simulink model "TaskB"  (R2022b)
settings: Solver=ode45  StartTime=0.0  StopTime=10.0  RelTol=1e-3
undefined symbols (not defined in the file): A_11, A_12, A_21, A_22, absolute_encoder_counts_per_revolution, B_1, B_2, init, K_I2, K_x2, L_d
libraries: simulink_extras x7
settings Model: Creator=tumisangramotlhwa  LastModifiedBy=tumisangramotlhwa

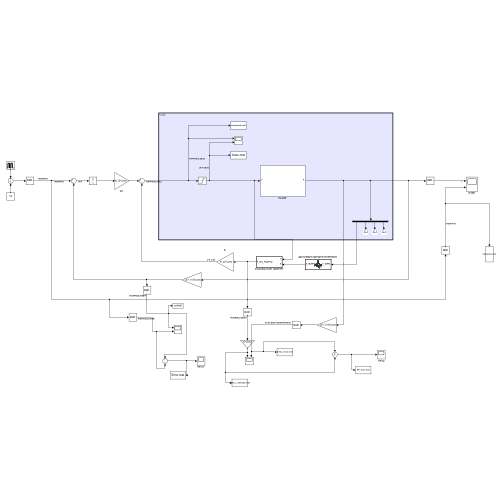
[thumbnail: Simulink's stored preview of the top-level diagram]
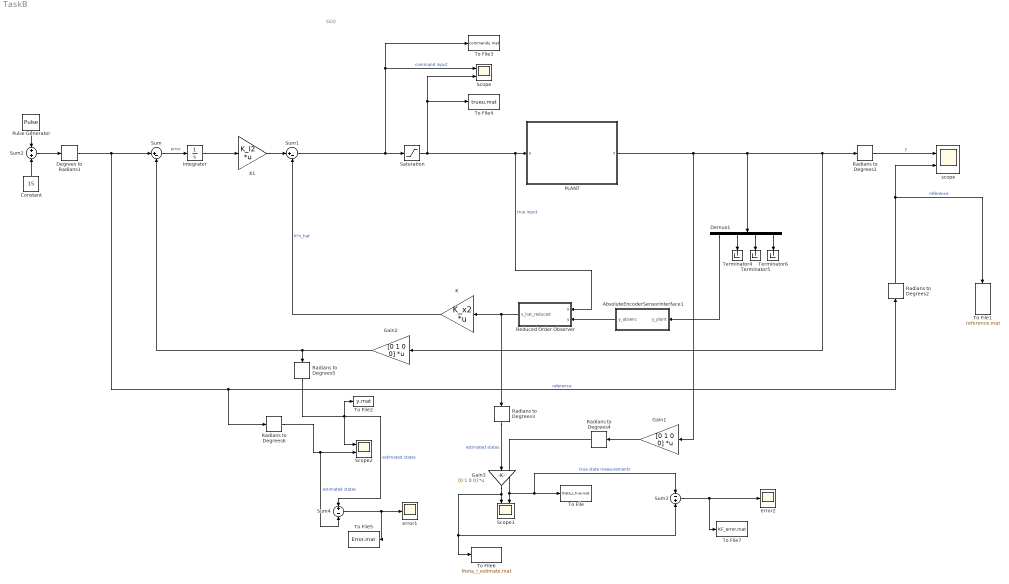
== system TaskB ==
  note: G(s)
  AbsoluteEncoderSensorInterface1 : Subsystem  TreatAsAtomicUnit=on
      mask Display: image('$imagefile'); % Use "Edit Image" on toolstrip to change.
  Constant : Constant  Value=15
  Degrees to Radians1 : simulink_extras/Transformations/Degrees to Radians
  Demux1 : Demux
  Gain1 : Gain  Gain=[0 1 0 0]  Multiplication=Matrix(K*u) (u vector)
  Gain2 : Gain  Gain=[0 1 0 0]  Multiplication=Matrix(K*u) (u vector)
  Gain3 : Gain  Gain=[0 1 0 0]  Multiplication=Matrix(K*u) (u vector)
  Integrator : Integrator
  K : Gain  Gain=K_x2  Multiplication=Matrix(K*u) (u vector)
  K1 : Gain  Gain=K_I2  Multiplication=Matrix(K*u) (u vector)
  PLANT : Subsystem
  Pulse Generator : DiscretePulseGenerator  PulseType=Time based  Amplitude=30  Period=4  PulseWidth=50
  Radians to Degrees{1..6} (6 alike) : simulink_extras/Transformations/Radians to Degrees
  Reduced Order Observer : Subsystem  TreatAsAtomicUnit=on
  Saturation : Saturate  UpperLimit=6  LowerLimit=-6
  Scope : Scope  NumInputPorts=2
  Scope1 : Scope  NumInputPorts=2
  Scope2 : Scope  NumInputPorts=2
  Sum : Sum  Inputs=|+-
  Sum1 : Sum  Inputs=|+-
  Sum2 : Sum  Inputs=+|+
  Sum3 : Sum  Inputs=-|+
  Sum4 : Sum  Inputs=+|-
  Terminator4 : Terminator
  Terminator5 : Terminator
  Terminator6 : Terminator
  To File : ToFile  Filename=theta_l_true.mat  MatrixName=theta_l_true  SaveFormat=Timeseries
  To File1 : ToFile  Filename=reference.mat  MatrixName=reference  SaveFormat=Timeseries
  To File2 : ToFile  Filename=y.mat  MatrixName=y  SaveFormat=Timeseries
  To File3 : ToFile  Filename=commandu.mat  MatrixName=commandu  SaveFormat=Timeseries
  To File4 : ToFile  Filename=trueu.mat  MatrixName=trueu  SaveFormat=Timeseries
  To File5 : ToFile  Filename=Error.mat  MatrixName=Error  SaveFormat=Timeseries
  To File6 : ToFile  Filename=theta_l_estimate.mat  MatrixName=theta_l_estimate  SaveFormat=Timeseries
  To File7 : ToFile  Filename=KF_error.mat  MatrixName=KF_error  SaveFormat=Timeseries
  error1 : Scope
  error2 : Scope
  scope : Scope  NumInputPorts=2
  wires:
  Pulse Generator/1 -> Sum2/1
  Saturation/1 -> Reduced Order Observer/1(u), PLANT/1(u), To File4/1, Scope/2  "true input"
  Integrator/1 -> K1/1
  Sum1/1 -> To File3/1, Scope/1, Saturation/1  "command input"
  K1/1 -> Sum1/1
  Sum2/1 -> Degrees to Radians1/1
  Constant/1 -> Sum2/2
  Radians to Degrees2/1 -> scope/2, To File1/1  "reference"
  K/1 -> Sum1/2  "K*x_hat"
  Radians to Degrees1/1 -> scope/1  "y"
  Degrees to Radians1/1 -> Radians to Degrees2/1, Radians to Degrees6/1, Sum/1  "reference"
  Sum/1 -> Integrator/1  "error"
  Reduced Order Observer/1(x_hat_reduced) -> K/1, Radians to Degrees3/1
  Radians to Degrees3/1 -> Gain3/1  "estimated states"
  Radians to Degrees4/1 -> Scope1/2, Sum3/1, To File/1  "true state measurements"
  AbsoluteEncoderSensorInterface1/1(y_absenc) -> Reduced Order Observer/2(y)
  Demux1/2 -> Terminator4/1
  Demux1/4 -> Terminator6/1
  Demux1/3 -> Terminator5/1
  PLANT/1(x) -> Gain2/1, Radians to Degrees1/1, Demux1/1, Gain1/1
  Demux1/1 -> AbsoluteEncoderSensorInterface1/1(y_plant)
  Gain2/1 -> Radians to Degrees5/1, Sum/2
  Radians to Degrees5/1 -> Scope2/1, Sum4/1, To File2/1  "estimated states"
  Radians to Degrees6/1 -> Sum4/2, Scope2/2  "estimated states"
  Sum4/1 -> To File5/1, error1/1
  Gain1/1 -> Radians to Degrees4/1
  Gain3/1 -> Sum3/2, To File6/1, Scope1/1
  Sum3/1 -> To File7/1, error2/1

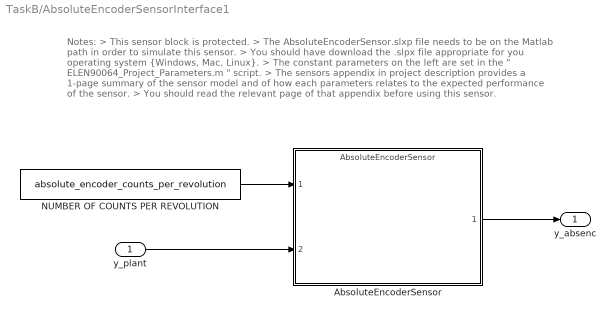
== system TaskB/AbsoluteEncoderSensorInterface1 ==
  note: Notes:
      | > This sensor block is protected.
      | > The AbsoluteEncoderSensor.slxp file needs to be on the Matlab path in order to simulate this sensor.
      | > You should have download the .slpx file appropriate for you operating system {Windows, Mac, Linux}.
      | > The constant parameters on the left are set in the " ELEN90064_Project_Parameters.m " script.
      | > The sensors appendix in project description provides a 1-page summary of the sensor model and of how each parameters relates to the expected performance of the sensor.
      | > You should read the relevant page of that appendix before using this sensor.
  y_plant : Inport
  AbsoluteEncoderSensor : ModelReference  ModelNameDialog=AbsoluteEncoderSensor.slxp  ModelReferenceVersion=1.16  CopyOfModelProtected=on
  NUMBER OF COUNTS PER REVOLUTION : Constant  Value=absolute_encoder_counts_per_revolution
  y_absenc : Outport
  wires:
  NUMBER OF COUNTS PER REVOLUTION/1 -> AbsoluteEncoderSensor/1
  y_plant/1 -> AbsoluteEncoderSensor/2
  AbsoluteEncoderSensor/1 -> y_absenc/1

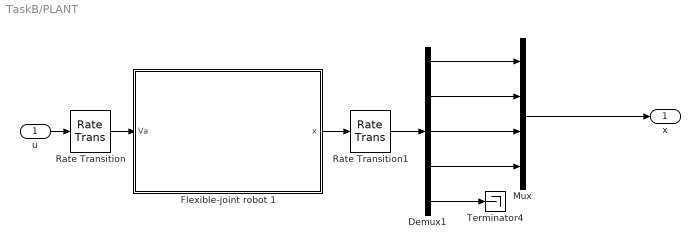
== system TaskB/PLANT ==
  u : Inport
  Demux1 : Demux  Outputs=5
  Flexible-joint robot 1 : Subsystem
      mask Display: image('$imagefile'); % Use "Edit Image" on toolstrip to change.
  Mux : Mux
  Rate Transition : RateTransition
  Rate Transition1 : RateTransition  OutPortSampleTime=Ts
  Terminator4 : Terminator
  x : Outport
  wires:
  Demux1/4 -> Mux/4
  Flexible-joint robot 1/1(x) -> Rate Transition1/1
  Demux1/3 -> Mux/3
  Demux1/2 -> Mux/2
  Demux1/1 -> Mux/1
  Demux1/5 -> Terminator4/1
  u/1 -> Rate Transition/1
  Rate Transition/1 -> Flexible-joint robot 1/1(Va)
  Mux/1 -> x/1
  Rate Transition1/1 -> Demux1/1

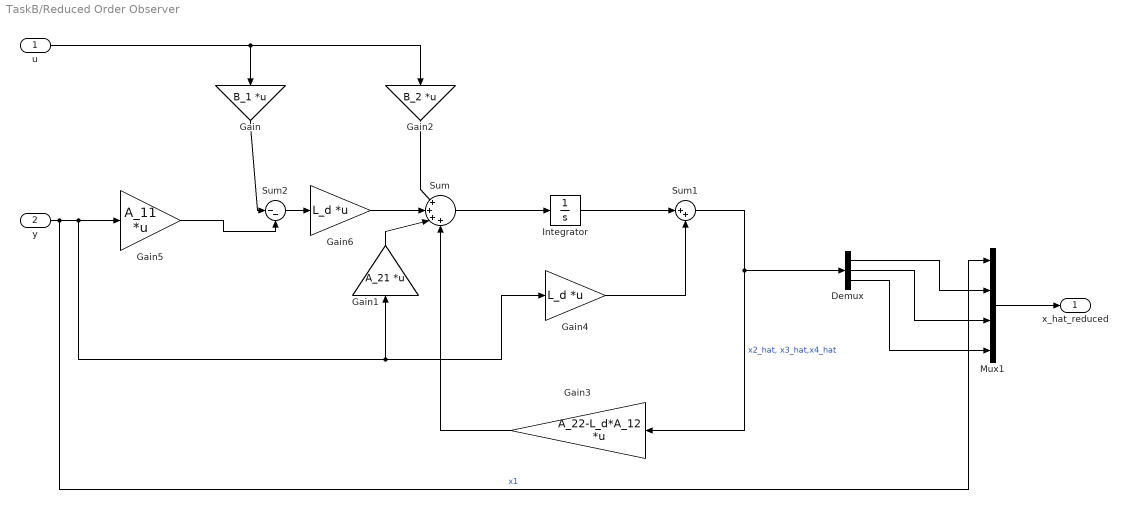
== system TaskB/Reduced Order Observer ==
  u : Inport
  y : Inport  Port=2
  Demux : Demux  Outputs=3
  Gain : Gain  Gain=B_1  Multiplication=Matrix(K*u) (u vector)
  Gain1 : Gain  Gain=A_21  Multiplication=Matrix(K*u) (u vector)
  Gain2 : Gain  Gain=B_2  Multiplication=Matrix(K*u) (u vector)
  Gain3 : Gain  Gain=A_22-L_d*A_12  Multiplication=Matrix(K*u) (u vector)
  Gain4 : Gain  Gain=L_d  Multiplication=Matrix(K*u) (u vector)
  Gain5 : Gain  Gain=A_11  Multiplication=Matrix(K*u) (u vector)
  Gain6 : Gain  Gain=L_d  Multiplication=Matrix(K*u) (u vector)
  Integrator : Integrator
  Mux1 : Mux
  Sum : Sum  Inputs=|++++
  Sum1 : Sum  Inputs=|++
  Sum2 : Sum  Inputs=|--
  x_hat_reduced : Outport
  wires:
  u/1 -> Gain2/1, Gain/1
  y/1 -> Mux1/1, Gain5/1, Gain4/1, Gain1/1  "x1"
  Sum/1 -> Integrator/1
  Gain6/1 -> Sum/2
  Gain1/1 -> Sum/3
  Gain/1 -> Sum2/1
  Gain5/1 -> Sum2/2
  Gain2/1 -> Sum/1
  Integrator/1 -> Sum1/1
  Gain4/1 -> Sum1/2
  Gain3/1 -> Sum/4
  Sum1/1 -> Demux/1, Gain3/1  "x2_hat, x3_hat,x4_hat"
  Sum2/1 -> Gain6/1
  Mux1/1 -> x_hat_reduced/1
  Demux/1 -> Mux1/2
  Demux/2 -> Mux1/3
  Demux/3 -> Mux1/4

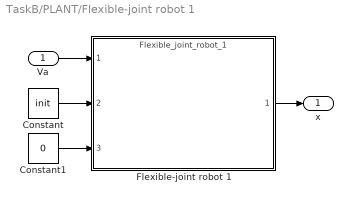
== system TaskB/PLANT/Flexible-joint robot 1 ==
  Va : Inport
  Constant : Constant  Value=init
  Constant1 : Constant  Value=0
  Flexible-joint robot 1 : ModelReference  ModelNameDialog=Flexible_joint_robot_1  ModelReferenceVersion=1.63  CopyOfModelProtected=on
  x : Outport
  wires:
  Constant/1 -> Flexible-joint robot 1/2
  Constant1/1 -> Flexible-joint robot 1/3
  Flexible-joint robot 1/1 -> x/1
  Va/1 -> Flexible-joint robot 1/1
